simulink model "SchemaPrincipala2"  (R2023b)
settings: Solver=VariableStepAuto  StartTime=0.0  StopTime=500  RelTol=1e-3
values from neighbouring files (symbols this model uses):
  a1 = 4.2175e-05    [matlab.mat]    (also in tema1.m)
  a2 = 4.4842e-05    [matlab.mat]    (also in tema1.m = 4.4841e-05)
  A2 = 0.021    [matlab.mat]    (also in tema1.m)
  ac = 4.307e-05    [matlab.mat]    (also in tema1.m = 4.307e-06)
  At = 0.1273    [matlab.mat]    (also in tema1.m)
  g = 9.8    [matlab.mat]    (also in tema1.m)
  H = 0.25    [matlab.mat]    (also in tema1.m)
  l = 0.14    [matlab.mat]    (also in tema1.m)
  L = 0.08    [matlab.mat]    (also in tema1.m)
  Q = 0.00011667    [matlab.mat]    (also in tema1.m)
  Qp1 = 5e-05    [matlab.mat]    (also in tema1.m)
  Qp2 = 5e-05    [matlab.mat]    (also in tema1.m)
  teta = 0.261666666667    [matlab.mat]    (also in tema1.m)
  u2 = 50/100    (= 0.5)    [tema1.m]
undefined symbols (not defined in the file or in its folder): u1
settings Model: Creator=Stefaneko  LastModifiedBy=Stefaneko

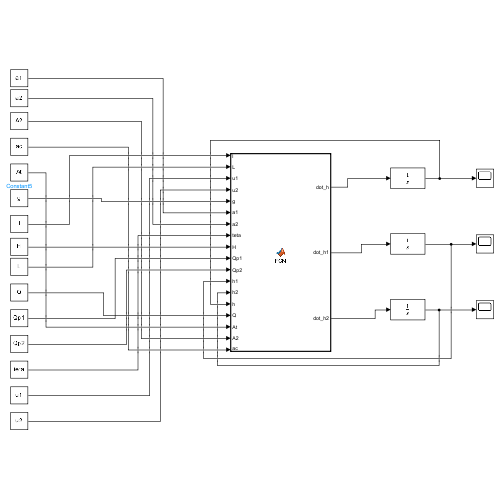
[thumbnail: Simulink's stored preview of the top-level diagram]
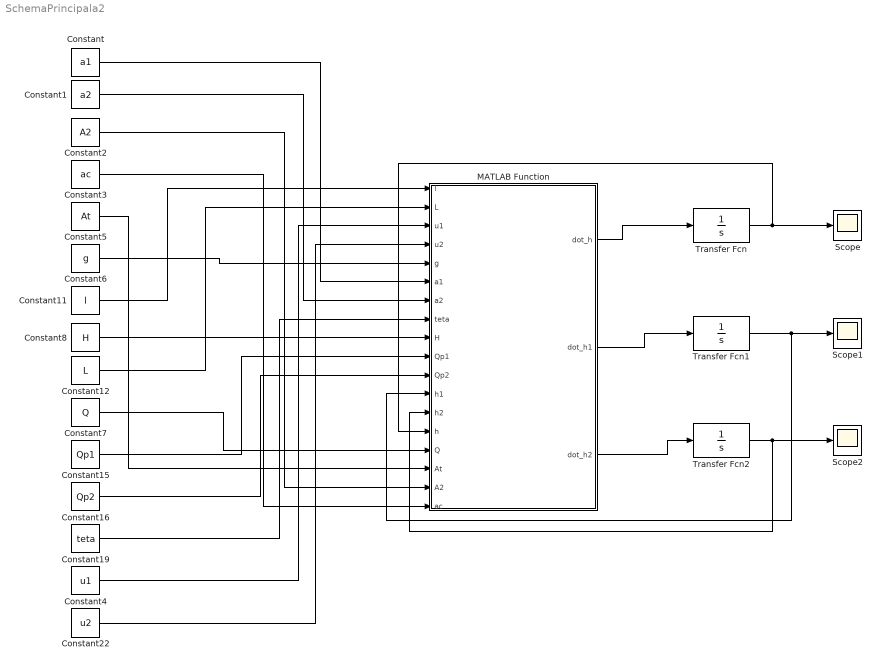
== system SchemaPrincipala2 ==
  Constant : Constant  Value=a1
  Constant1 : Constant  Value=a2
  Constant11 : Constant  Value=l
  Constant12 : Constant  Value=L
  Constant15 : Constant  Value=Qp1
  Constant16 : Constant  Value=Qp2
  Constant19 : Constant  Value=teta
  Constant2 : Constant  Value=A2
  Constant22 : Constant  Value=u2
  Constant3 : Constant  Value=ac
  Constant4 : Constant  Value=u1
  Constant5 : Constant  Value=At
  Constant6 : Constant  Value=g
  Constant7 : Constant  Value=Q
  Constant8 : Constant  Value=H
  MATLAB Function : MATLAB Function  TreatAsAtomicUnit=on
  Scope : Scope
  Scope1 : Scope
  Scope2 : Scope
  Transfer Fcn : TransferFcn  Denominator=[1 0]
  Transfer Fcn1 : TransferFcn  Denominator=[1 0]
  Transfer Fcn2 : TransferFcn  Denominator=[1 0]
  wires:
  Constant6/1 -> MATLAB Function/5(g)
  Constant16/1 -> MATLAB Function/11(Qp2)
  Constant15/1 -> MATLAB Function/10(Qp1)
  Constant3/1 -> MATLAB Function/18(ac)
  Constant11/1 -> MATLAB Function/1(l)
  Constant12/1 -> MATLAB Function/2(L)
  MATLAB Function/1(dot_h) -> Transfer Fcn/1
  MATLAB Function/2(dot_h1) -> Transfer Fcn1/1
  MATLAB Function/3(dot_h2) -> Transfer Fcn2/1
  Transfer Fcn/1 -> Scope/1, MATLAB Function/14(h)
  Transfer Fcn1/1 -> Scope1/1, MATLAB Function/12(h1)
  Transfer Fcn2/1 -> Scope2/1, MATLAB Function/13(h2)
  Constant/1 -> MATLAB Function/6(a1)
  Constant1/1 -> MATLAB Function/7(a2)
  Constant7/1 -> MATLAB Function/15(Q)
  Constant5/1 -> MATLAB Function/16(At)
  Constant2/1 -> MATLAB Function/17(A2)
  Constant4/1 -> MATLAB Function/3(u1)
  Constant22/1 -> MATLAB Function/4(u2)
  Constant19/1 -> MATLAB Function/8(teta)
  Constant8/1 -> MATLAB Function/9(H)

== matlab function SchemaPrincipala2/MATLAB Function ==
  data: l input; L input; u1 input; u2 input; g input; a1 input; a2 input; teta input; H input; Qp1 input; Qp2 input; h1 input; h2 input; h input; Q input; At input; A2 input; dot_h output; ac input; dot_h1 output; dot_h2 output
function [dot_h,dot_h1,dot_h2] = FCN(l,L,u1,u2,g,a1,a2,teta,H,Qp1,Qp2,h1,h2,h, Q, At, A2, ac)
u11=u1*5;
u22=u2*5;
dot_h1=1/(l*(L+h1*tan(teta)))*((((u1/(u1+u2))*((u1+u2)/100)/2)*Q+u11*Qp1-a1*sqrt(abs(2*(g*h1*(1+(h1/(4*L))*sin(2*teta))-g*H*H/(4*L)*sin(2*teta)))))-ac*sign(h1-h2+((h1*H)/2*L)*sin(2*teta)-(H*H)/(4*L)*sin(2*teta))*sqrt(abs(2*g*abs(h1-h2+((h1*H)/2*L)*sin(2*teta)-(H*H)/(4*L)*sin(2*teta)))));
dot_h2=(1/A2)*(((u2/(u1+u2))*((u1+u2)/100)/2)*Q+u22*Qp2-a2*sqrt(abs(2*g*h2))+ac*sign(h1-h2+((h1*H)/(2*L)*sin(2*teta)-(H*H)/(4*L)*sin(2*teta))*sqrt(abs(2*g*abs(h1-h2+((h1*H)/2*L)*sin(2*teta)-(H*H)/(4*L)*sin(2*teta))))));
dot_h=(1/At)*(a1*sqrt(abs(2*(g*h1*(1+(H/(2*L))*sin(2*teta)))-g*H*H/(2*L)*sin(2*teta)))+a2*sqrt(abs(2*g*h2))-u11*Qp1-u22*Qp2);
